simulink model "LQR_ACC_Current"  (R2024a)
settings: Solver=FixedStepAuto  StartTime=0  StopTime=1000  FixedStep=0.05  RelTol=1e-3
undefined symbols (not defined in the file or in its folder): acc_max, acc_min, Defined, driver_set_speed, Ego, jerk_lim, K_derr, K_vh, Lane, matlabshared, preview_time_AEB, preview_time_set_spd, rel_vel_thresh, rho, simStepSize, User
libraries: roadrunnerscenario x4, dsa_UDP_Blockset x2, drivingscenarioandsensors x1, autolibshared x1
settings Model: PacingRate=10  Creator=darkh  LastModifiedBy=darkh
settings DataIOCC: ReturnWorkspaceOutputsName=sltest_internal_rrSimulationOutputVariable
settings DebuggingCC: AlgebraicLoopMsg=none
settings RTWCC: GPUComputeCapability=3.5
settings ConfigComp: CovSaveName=sltest_covdata  CovMetricSettings=dcmwe  CovEnableCumulative=off  CovSaveSingleToWorkspaceVar=on  CovSaveOutputData=off

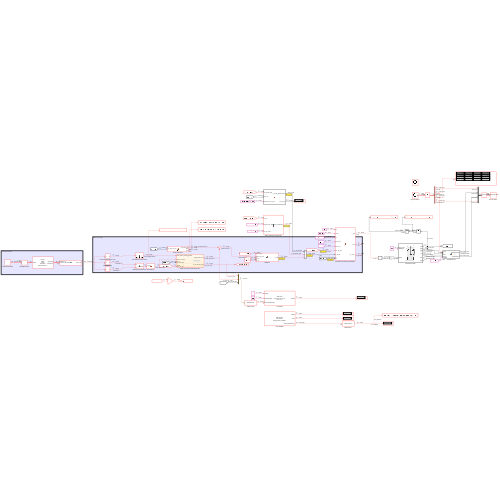
[thumbnail: Simulink's stored preview of the top-level diagram]
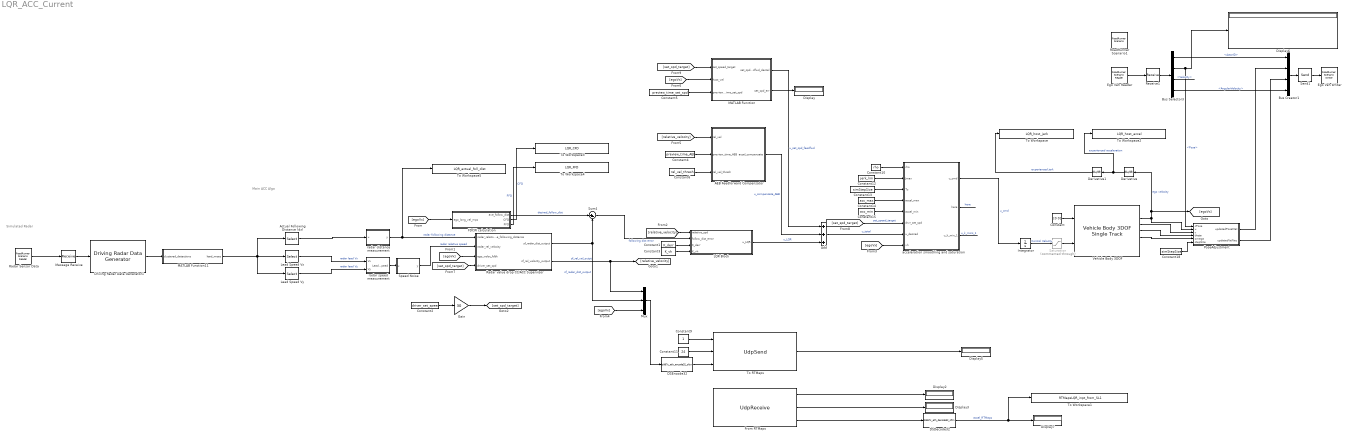
== system LQR_ACC_Current ==
  note: Simulated Radar
  note: Main ACC Algo
  AEB Feedforward Compensator : MATLAB Function  TreatAsAtomicUnit=on
  Actual Following Distance (dx) : Selector  InputPortWidth=6  IndexOptions=Index vector (dialog)  Indices=[1]  OutputSizes=1
  Add : Sum  Inputs=+++
  Bus Creator1 : BusCreator  Inputs=4  OutDataTypeStr=Bus: BusActorRuntime  NonVirtualBus=on
      settings: InheritFromInputs=off
  Bus Selector3 : BusSelector  OutputSignals=ActorID,Pose,Velocity,AngularVelocity
  Constant : Constant  Value=[0 0]
  Constant1 : Constant  Value=K_derr  SampleTime=simStepSize
  Constant10 : Constant  Value=rho
  Constant11 : Constant  Value=24
  Constant12 : Constant  Value=jerk_lim
  Constant13 : Constant  Value=simStepSize
  Constant14 : Constant  Value=acc_max
  Constant15 : Constant  Value=acc_min
  Constant18 : Constant  Value=simStepSize
  Constant2 : Constant  Value=driver_set_speed  SampleTime=simStepSize
  Constant3 : Constant  Value=K_vh  SampleTime=simStepSize
  Constant4 : Constant  Value=preview_time_AEB
  Constant5 : Constant  Value=preview_time_set_spd
  Constant6 : Constant  Value=rel_vel_thresh
  Constant9 : Constant
  "DSDecode32 " : S-Function  FunctionName=ds867c_eth_decode32_sfcn  Parameters=byteordering,offset,auto_offset,datatype,one_datatype,sampletime  SFunctionDeploymentMode=off  EnableBusSupport=off  mask(DSDecode32){byteordering=big endian (Motorola), offset=[0], auto_offset=on, datatype=[9], one_datatype=off, sampletime=-1}
      mask prompts: byteordering "Byte ordering:"; offset "Offset (bytes):"; auto_offset "Auto offset"; one_datatype "One datatype only"
      mask help:
      | Converts a 32bit WORD input data stream into the specified datatypes on the output port.
      |
      | Datatype Codes:
      | BOOLEAN:  1   //   INT8      :  2    //   UINT8    :  3
      | INT16       :  4   //   UINT16 :  5    //   INT32     :  6
      | UINT32    :  7   //   FLOAT   :  8    //   DOUBLE:  9
      mask Help:
      | The 'DSDecode32' block allows to decode an UInt32 vector containing encoded elements of various data types to an output vector of double values. It is intended to use this block in conjunction with the 'DS4504_ETH_Receive' block which delivers this format as data output. Data received from the Ethernet via the 'DS4504_ETH_Receive' block is performed in Intel byte order ('Little Endian').
      | 
      | <br>
      | <br>
      | 
      | <h2>Parameters</h2>
      | <br>
      | <br>
      | 
      | <b>Byte ordering (only relevant for offline simulation)</b>
      | <br>
      | <blockquote>
      | The byte order of the input vector has to be specified. In case of running a real-time application the appropriate byte order (Motorola for DS1005 and Intel for DS1006) is selected automatically. Therefore the byte order setting has no influence on the online simulation.
      | </blockquote>
      | <br>
      | 
      | <b>Offset (bytes)</b>
      | <br>
      | <blockquote>
      | This is for defining a vector of offsets which specifies the position of each element within the input vector. The offsets must be entered as an array (e.g. [1 10 . 50 54] ) using the same order as for the corresponding data type vector (see (4)). This option is useful if you have gaps between adjacent elements.
      | </blockquote>
      | <br>
      | 
      | <b>Auto offset</b>
      | <br>
      | <blockquote>
      | When activating this checkbox parameter, the edit field 'Offset' is disabled and the byte offsets in the input vector are calculated automatically concerning the specified data types (no gaps presupposed). Any previous setting in the offset vector would be ignored.
      | </blockquote>
      | <br>
      | 
      | <b>Datatype</b>
      | <br>
      | <blockquote>
      | This is for defining a vector of data types which specifies the type for each element in the input vector. Supported data types are Boolean, Int8, UInt8, Int16, UInt16, Int32, UInt32, Float and Double, which are determined by using the corresponding data type codes shown in the following table:
      | <br>
      | <br>
      | <table BORDER=1 ALIGN="center">
      | <TR>
      | <TH WIDTH=20%>Data type</TH>
      | <TH WIDTH=20%>Data type code</TH>
      | <TH WIDTH=20%>Length in bytes</TH>
      | </TR>
      | <TR><TD>Boolean</TD><TD ALIGN="center">1</TD><TD ALIGN="center">1</TD></TR>
      | <TR><TD>Int8</TD><TD ALIGN="center">2</TD><TD ALIGN="center">1</TD></TR>
      | <TR><TD>Uint8</TD><TD ALIGN="center">3</TD><TD ALIGN="center">1</TD></TR>
      | <TR><TD>Int16</TD><TD ALIGN="center">4</TD><TD ALIGN="center">2</TD></TR>
      | <TR><TD>Uint16</TD><TD ALIGN="center">5</TD><TD ALIGN="center">2</TD></TR>
      | <TR><TD>Int32</TD><TD ALIGN="center">6</TD><TD ALIGN="center">4</TD></TR>
      | <TR><TD>Uint32</TD><TD ALIGN="center">7</TD><TD ALIGN="center">4</TD></TR>
      | <TR><TD>Float</TD><TD ALIGN="center">8</TD><TD ALIGN="center">4</TD></TR>
      | <TR><TD>Double</TD><TD ALIGN="center">9</TD><TD ALIGN="center">8</TD></TR>
      | </TABLE>
      | </blockquote>
      | <br>
      | 
      | <b>One datatype only</b>
      | <br>
      | <blockquote>
      | This option is useful if all elements of the input vector have the same data type. If the checkbox is activated the first element of the data type vector specifies the data type to be used. In this case it is naturally sufficient to enter only one number which applies for the complete input vector.
      | </blockquote>
      | <br>
      | 
      | <b>Sample time</b>
      | <br>
      | <blockquote>
      | The desired sample time for this block has to be entered here. Alternatively it can be  inherited from the Simulink model by using '-1'.
      | </blockquote>
      | <br>
      mask TypeOptions byteordering: big endian (Motorola) | little endian (Intel)
      mask Display: text(0.5,0.5,'DSDecode32','HorizontalAlignment','center')
  DSEncode32 : S-Function  FunctionName=ds867c_eth_encode32_sfcn  Parameters=byteordering,offset,auto_offset,datatype,one_datatype,sampletime  SFunctionDeploymentMode=off  EnableBusSupport=off  mask(DSEncode32){byteordering=big endian (Motorola), offset=[ 0 ], auto_offset=on, datatype=[9,9,9], one_datatype=off, sampletime=-1}
      mask prompts: byteordering "Byte ordering:"; offset "Offset (bytes):"; auto_offset "Auto offset"; one_datatype "One datatype only"
      mask help:
      | Converts an input signal consisting of datatypes into a 32Bit WORD data stream on the output port.
      |
      | Datatype Codes:
      | BOOLEAN:  1   //   INT8      :  2    //   UINT8    :  3
      | INT16       :  4   //   UINT16 :  5    //   INT32     :  6
      | UINT32    :  7   //   FLOAT   :  8    //   DOUBLE:  9
      mask Help:
      | The 'DSEncode32' block is responsible for converting the input vector consisting of double values to different data types (multi-byte numbers) and merging them into a data stream composed of an array of UInt32 variables. It is intended to use this block in conjunction with the 'DS4504_ETH_Send' block which delivers the data in Intel byte order to the network.
      | 
      | <br>
      | <br>
      | 
      | <h2>Parameters</h2>
      | <br>
      | <br>
      | 
      | <b>Byte ordering (only relevant for offline simulation)</b>
      | <br>
      | <blockquote>
      | It lets the user choose the byte order (Motorola or Intel) of the output vector. The way multibyte numbers (e.g. Float = 4 bytes or Int16 = 2 bytes) are stored in memory depends on the used computing system. There are two possible formats which are called "Little Endian" and "Big Endian". "Little Endian" means that the low-order byte of the number is stored at the lowest and the high-order byte at the highest memory address. "Big Endian" means the opposite.
      | This option is only relevant for offline (Simulink) simulation. In case of running a real-time application the appropriate byte order (Motorola for DS1005 and Intel for DS1006) is selected automatically. Therefore the byte order setting has no influence on the online simulation.
      | </blockquote>
      | <br>
      | 
      | <b>Offset (bytes)</b>
      | <br>
      | <blockquote>
      | This is for defining a vector of offsets which specifies the position of each input element within the output byte vector. The offsets must be entered as an array (e.g. [1 10 . 50 54] ) using the same order as for the corresponding data type vector (see (4)). This option is useful if you want to have gaps between adjacent elements (e.g. in order to avoid access to even bytes).
      | <br>
      | <br>
      | <i>Important Note:</i>
      | <br>
      | By means of the offset vector the specified data values can be located flexibly within the UInt32 word stream, presupposed that the data values do not overlap. Otherwise data loss occurs.
      | </blockquote>
      | <br>
      | 
      | <b>Auto offset</b>
      | <br>
      | <blockquote>
      | When activating this checkbox parameter, the edit field 'Offset' is disabled and the required byte offsets for the input data types will be calculated automatically without gaps (for tight packing). This option is always useful if there is no need for special offsets (no gaps between two adjacent elements). Any previous setting in the offset vector would be ignored.
      | </blockquote>
      | <br>
      | 
      | <b>Datatype</b>
      | <br>
      | <blockquote>
      | This is for defining a vector of data types which specifies the type for each input element in the output byte vector. Supported data types are Boolean, Int8, UInt8, Int16, UInt16, Int32, UInt32, Float and Double, which are determined by using the corresponding data type codes shown in the following table:
      | <br>
      | <br>
      | <table BORDER=1 ALIGN="center">
      | <TR>
      | <TH WIDTH=20%>Data type</TH>
      | <TH WIDTH=20%>Data type code</TH>
      | <TH WIDTH=20%>Length in bytes</TH>
      | </TR>
      | <TR><TD>Boolean</TD><TD ALIGN="center">1</TD><TD ALIGN="center">1</TD></TR>
      | <TR><TD>Int8</TD><TD ALIGN="center">2</TD><TD ALIGN="center">1</TD></TR>
      | <TR><TD>Uint8</TD><TD ALIGN="center">3</TD><TD ALIGN="center">1</TD></TR>
      | <TR><TD>Int16</TD><TD ALIGN="center">4</TD><TD ALIGN="center">2</TD></TR>
      | <TR><TD>Uint16</TD><TD ALIGN="center">5</TD><TD ALIGN="center">2</TD></TR>
      | <TR><TD>Int32</TD><TD ALIGN="center">6</TD><TD ALIGN="center">4</TD></TR>
      | <TR><TD>Uint32</TD><TD ALIGN="center">7</TD><TD ALIGN="center">4</TD></TR>
      | <TR><TD>Float</TD><TD ALIGN="center">8</TD><TD ALIGN="center">4</TD></TR>
      | <TR><TD>Double</TD><TD ALIGN="center">9</TD><TD ALIGN="center">8</TD></TR>
      | </TABLE>
      | </blockquote>
      | <br>
      | 
      | <b>One datatype only</b>
      | <br>
      | <blockquote>
      | This option is useful if all elements of the data input vector shall be converted to the same data type in the output vector. If the checkbox is activated the first element of the data type vector specifies the data type to be used. In this case it is naturally sufficient to enter only one number which applies for the complete input vector.
      | </blockquote>
      | <br>
      | 
      | <b>Sample time</b>
      | <br>
      | <blockquote>
      | The desired sample time for this block has to be entered here. Alternatively it can be  inherited from the Simulink model by using '-1'.
      | </blockquote>
      | <br>
      mask TypeOptions byteordering: big endian (Motorola) | little endian (Intel)
      mask Display: text(0.5,0.5,'DSEncode32','HorizontalAlignment','center')
  Derivative : Derivative
  Derivative1 : Derivative
  Display{,2..3,5..7} (6 alike) : Display
  Driving Radar Data Generator1 : drivingscenarioandsensors/Driving Radar Data Generator  SensorIndex=1  UpdateRate=20  MountingLocation=[ 3.4, 0, 0.2 ]  MountingAngles=[0 0 0]  HasElevation=off  HasRangeRate=on  HasNoise=off  HasFalseAlarms=off  HasOcclusion=off  MaxNumReportsSource=Property  MaxNumReports=50  TargetReportFormat=Clustered detections  DetectionCoordinates=Body  TrackCoordinates=Body  BusNameSource=Auto  BusName=BusDrivingRadarDataGenerator  AzimuthResolution=4  ElevationResolution=5  RangeResolution=2.5  RangeRateResolution=0.05  AzimuthBiasFraction=0.1  ElevationBiasFraction=0.1  RangeBiasFraction=0.01  RangeRateBiasFraction=0.01  FieldOfView=[ 20, 5 ]  RangeLimits=[ 0, 150 ]  RangeRateLimits=[ -100, 100 ]  DetectionProbability=1  FalseAlarmRate=1e-06  ReferenceRange=100  ReferenceRCS=0  CenterFrequency=77e9  FilterInitializationFcn=initcvekf  ConfirmationThreshold=[2 3]  DeletionThreshold=[5 5]  InitialSeedSource=Repeatable  InitialSeed=0  UsedSeed=matlabshared.tracking.internal.SimulinkUtilities.seedManager(gcb)  ProfilesSource=From Scenario Reader block  ProfilesParameters=driving.internal.ActorProfilesRadarParameters  ProfilesExpression=struct('ClassID',0,'Length',4.7,'Width',1.8,'Height',1.4,'OriginOffset',[-1.35 0 0],'RCSPattern',[10 10;10 10],'RCSAzimuthAngles',[-180 180],'RCSElevationAngles',[-90 90])
  Ego Veh Reader : roadrunnerscenario/RoadRunner Scenario Reader  TopicCategory=Actor  ActorCategory=All Types  ActionType=Path Following  EventType=User-Defined  TopicType=Actor Pose  VehicleType=Vehicle Specifications  UserDefinedAction=Action1  UserDefinedEvent=Event1  Filter=Self  SensorTopic=Target Poses  LaneBoundaryOutputTopic=Ego-Lane  SensorID=1  SampleTime=simStepSize
  Ego Veh Writer : roadrunnerscenario/RoadRunner Scenario Writer  TopicCategory=Actor  ActorCategory=All Types  EventType=Action Complete  UserDefinedEvent=Event1  VehicleType=Vehicle Pose  TopicType=Actor Pose
  FDCW calculation : MATLAB Function  TreatAsAtomicUnit=on
  From RTMaps : dsa_UDP_Blockset/UdpReceive  portNumber=25000  sampleTime=simStepSize  outputWidth=1472  rxTimeout=1  rxBufferSize=73600
  Gain : Gain  Gain=30
  Integrator : Integrator
  LQR Block : MATLAB Function  TreatAsAtomicUnit=on  SystemSampleTime=simStepSize
  Lead Speed Vx : Selector  InputPortWidth=6  IndexOptions=Index vector (dialog)  Indices=4  OutputSizes=1
  Lead Speed Vy : Selector  InputPortWidth=6  IndexOptions=Index vector (dialog)  Indices=5  OutputSizes=1
  MATLAB Function : MATLAB Function  TreatAsAtomicUnit=on
  MATLAB Function11 : MATLAB Function  TreatAsAtomicUnit=on
  Message Receive : Receive  InputPortMessageModes=m  UseInternalQueue=off
  Mux : Mux  Inputs=3
  PoseAdjustment : MATLAB Function  TreatAsAtomicUnit=on
  Radar Sensor Data : roadrunnerscenario/RoadRunner Scenario Reader  TopicCategory=Sensor  ActorCategory=All Types  ActionType=Path Following  EventType=User-Defined  TopicType=Actor Specifications  VehicleType=Vehicle Specifications  UserDefinedAction=Action1  UserDefinedEvent=Event1  Filter=Self  SensorTopic=Target Poses  LaneBoundaryOutputTopic=Ego-Lane  SensorID=1  SampleTime=simStepSize
  Radar value drop CC/ACC Supervisor : Stateflow chart  TreatAsAtomicUnit=on
  Receive1 : Receive  InputPortMessageModes=m  UseInternalQueue=off  QueueOverwriting=on  QueueLength=1  QueueType=LIFO
  RoadRunner Scenario1 : roadrunnerscenario/RoadRunner Scenario  UserDefinedActions={}  UserDefinedEvents={}
  Saturation : Saturate  Commented=through  UpperLimit=driver_set_speed  LowerLimit=0
  Send1 : Send  OutputPortMessageModes=m
  Speed Noise : MATLAB Function  TreatAsAtomicUnit=on
  Sum4 : Sum  Inputs=|+-
  To RTMaps : dsa_UDP_Blockset/UdpSend  hostName=192.168.140.10  portNumber=11111
  To Workspace : ToWorkspace  VariableName=LQR_host_jerk  SampleTime=-1
  To Workspace1 : ToWorkspace  VariableName=RTMapsLQR_inpt_from_SL1  SaveFormat=Timeseries  SampleTime=-1
  To Workspace2 : ToWorkspace  VariableName=LQR_host_accel  SampleTime=-1
  To Workspace3 : ToWorkspace  VariableName=LQR_CFD  SampleTime=-1
  To Workspace4 : ToWorkspace  VariableName=LQR_FFD  SampleTime=-1
  To Workspace5 : ToWorkspace  VariableName=LQR_actual_foll_dist  SampleTime=-1
  "Vehicle Body 3DOF " : autolibshared/Vehicle Body 3DOF Single Track  trackMode=Dual  inputMode=External longitudinal velocity  frontSteerMode=on  rearSteerMode=off  windMode=off  muMode=off  extFMode=off  extMMode=off  htchFMode=off  htchMMode=off  extXo=off  extpsio=off  extxdoto=off  extro=off  extYo=off  extTamb=off  extydoto=off  aMode=2  NF=2  NR=2  m=2630.84  a=1.5569  b=1.5371  h=0.18903  dh=1  hh=0.2  X_o=0  xdot_o=0  CalphaMode=off  sigmaMode=on  d=0  hl=0  w=[1.4,1.4]  Cy_f=40000  Cy_r=40000  sigma_f=.1  sigma_r=.1  alpha_f_brk=[-.1 .1]  Cy_f_data=[-9e3 9e3]  alpha_r_brk=[-.1 .1]  Cy_r_data=[-9e3 9e3]  Y_o=0  ydot_o=0  Izz=2066  psi_o=0  r_o=0  Af=2.73  Cd=.30356  Cl=.1  Cpm=.1  beta_w=[0 0.01:0.01:0.3]  Cs=[0 0.01:0.01:0.3]  Cym=[0 1e-6:0.01:0.3]  Pabs=101325  Tair=273  g=9.81  mu=1  xdot_tol=.01  Fznom=5000  Fxtire_sat=7e4  Fytire_sat=7e4  longOff=0  latOff=0  vertOff=0  wrapAng=off
  acceleration smoothing and saturation : MATLAB Function  TreatAsAtomicUnit=on  SystemSampleTime=simStepSize
  radar distance measurement : MATLAB Function  TreatAsAtomicUnit=on
  radar speed measurement : MATLAB Function  TreatAsAtomicUnit=on
  wires:
  Bus Selector3/4 -> Bus Creator1/4  "<AngularVelocity>"
  Bus Creator1/1 -> Send1/1
  Bus Selector3/1 -> Bus Creator1/1  "<ActorID>"
  Receive1/1 -> Bus Selector3/1
  Send1/1 -> Ego Veh Writer/1
  Ego Veh Reader/1 -> Receive1/1
  "Vehicle Body 3DOF "/3 -> PoseAdjustment/3(v)
  "Vehicle Body 3DOF "/4 -> PoseAdjustment/4(theta)
  "Vehicle Body 3DOF "/5 -> PoseAdjustment/5(omega)
  Bus Selector3/2 -> Display6/1, PoseAdjustment/1(cPose)  "<Pose>"
  PoseAdjustment/1(updatedPoseMat) -> Bus Creator1/2
  "Vehicle Body 3DOF "/2 -> PoseAdjustment/2(u), Derivative/1, [egoVx]  "ego velocity"
  Radar Sensor Data/1 -> Message Receive/1
  Message Receive/1 -> Driving Radar Data Generator1/1
  Driving Radar Data Generator1/1 -> MATLAB Function11/1(clustered_detections)
  PoseAdjustment/2(updatedVelVec) -> Bus Creator1/3
  Integrator/1 -> Saturation/1  "Control Velocity"
  Constant/1 -> "Vehicle Body 3DOF "/1
  Sum4/1 -> LQR Block/2(follow_dist_error)  "following dist error"
  Constant1/1 -> LQR Block/3(K_derr)
  Lead Speed Vx/1 -> radar speed measurement/1(Vx)  "radar lead Vx"
  [egoVx] -> FDCW calculation/1(ego_long_vel_mps)
  FDCW calculation/1(ave_follow_dist) -> Sum4/1  "desired_follow_dist"
  MATLAB Function11/1(lead_meas) -> Actual Following Distance (dx)/1, Lead Speed Vy/1, Lead Speed Vx/1
  Lead Speed Vy/1 -> radar speed measurement/2(Vy)  "radar lead Vy"
  radar speed measurement/1(LeadSpeed) -> Speed Noise/1(u)
  FDCW calculation/2(CFD) -> To Workspace3/1  "CFD"
  Actual Following Distance (dx)/1 -> radar distance measurement/1(u)
  Derivative/1 -> To Workspace2/1, Derivative1/1  "experienced acceleration"
  Derivative1/1 -> To Workspace/1  "experienced jerk"
  [egoVx] -> Radar value drop CC/ACC Supervisor/3(ego_veloc_fdbk)
  Constant2/1 -> Gain/1
  Speed Noise/1(y) -> Radar value drop CC/ACC Supervisor/2(radar_rel_velocity)  "radar relative speed"
  radar distance measurement/1(y) -> To Workspace5/1, Radar value drop CC/ACC Supervisor/1(radar_relative_following_distance)  "radar following distance"
  Radar value drop CC/ACC Supervisor/1(sf_radar_dist_output) -> Mux/2, Sum4/2  "sf_radar_dist_output"
  Radar value drop CC/ACC Supervisor/2(sf_rel_velocity_output) -> Mux/1, [relative_velocity]  "sf_rel_vel_outpt"
  Constant3/1 -> LQR Block/4(K_vh)
  Mux/1 -> DSEncode32/1
  Constant9/1 -> To RTMaps/1
  Constant11/1 -> To RTMaps/2
  To RTMaps/1 -> Display5/1
  From RTMaps/1 -> Display2/1
  From RTMaps/2 -> Display3/1
  From RTMaps/3 -> "DSDecode32 "/1
  DSEncode32/1 -> To RTMaps/3
  "DSDecode32 "/1 -> Display7/1, To Workspace1/1  "accel_RTMaps"
  LQR Block/1(u_LQR) -> Add/3  "u_LQR"
  Constant12/1 -> acceleration smoothing and saturation/2(Jmax)
  Constant13/1 -> acceleration smoothing and saturation/3(Ts)
  Constant14/1 -> acceleration smoothing and saturation/4(accel_max)
  Constant15/1 -> acceleration smoothing and saturation/5(accel_min)
  Constant10/1 -> acceleration smoothing and saturation/1(rho)
  [egoVx] -> acceleration smoothing and saturation/8(vh)
  [set_spd_target] -> acceleration smoothing and saturation/6(drvr_set_spd)  "set_speed_target"
  Bus Selector3/3 -> ?  "<Velocity>"
  Saturation/1 -> "Vehicle Body 3DOF "/2
  [egoVx] -> Mux/3
  FDCW calculation/3(FFD) -> To Workspace4/1  "FFD"
  acceleration smoothing and saturation/1(u_cmd) -> Integrator/1  "u_cmd"
  Constant18/1 -> PoseAdjustment/6(stepSize)
  [relative_velocity] -> LQR Block/1(relative_spd)
  [relative_velocity] -> AEB Feedforward Compensator/1(rel_vel)
  Constant4/1 -> AEB Feedforward Compensator/2(preview_time_AEB)
  Constant6/1 -> AEB Feedforward Compensator/3(rel_vel_thresh)
  AEB Feedforward Compensator/1(accel_compensate) -> Add/2  "u_compensate_AEB"
  Add/1 -> acceleration smoothing and saturation/7(u_desired)  "u_total"
  MATLAB Function/2(set_spd_err) -> Display/1
  [egoVx] -> MATLAB Function/2(host_vel)
  Constant5/1 -> MATLAB Function/3(preview_time_set_spd)
  MATLAB Function/1(set_spd_feedfwd_deccel) -> Add/1  "u_set_spd_feedfwd"
  [set_spd_target] -> Radar value drop CC/ACC Supervisor/4(driver_set_spd)
  [set_spd_target] -> MATLAB Function/1(set_speed_target)
  Gain/1 -> [set_spd_target]
  acceleration smoothing and saturation/2(here) -> ?  "here"
  acceleration smoothing and saturation/3(u_k_min_1) -> ?  "u_k_mins_1"

== matlab function LQR_ACC_Current/radar distance measurement ==
  data: u input; y output
function y = removeSpikes(u)

    persistent buffer;
    persistent bufferIndex;
    threshold = 2;
    windowSize = 15;
    % windowSize = 4;
    
    if isempty(buffer)
        buffer = zeros(1, windowSize);
        bufferIndex = 1;
    end
    
    % Update buffer with new value
    buffer(bufferIndex) = u;
    bufferIndex = mod(bufferIndex, windowSize) + 1;
    
    % Calculate the median of the buffer
    medVal = median(buffer);
    
    % Detect and remove spikes
    if abs(u - medVal) > threshold
        y = medVal; % Replace spike with the median value
    else
        y = u; % Keep the original value if it's not a spike
    end
end

== matlab function LQR_ACC_Current/radar speed measurement ==
  data: Vx input; LeadSpeed output; Vy input
function LeadSpeed = fcn(Vx, Vy)

if Vx == 0 && Vy == 0 
    Vx = 0.01;
    Vy = 0.01;
elseif Vy == 0
    Vy = 0.01;
elseif Vx == 0
    Vx = 0.01;
end

if Vx <= 0
    LeadSpeed = -sqrt(Vx^2 + Vy^2);
else
    LeadSpeed = sqrt(Vx^2 + Vy^2);
end

== matlab function LQR_ACC_Current/Speed Noise ==
  settings: updateMethod=DISCRETE
  data: u input; y output
function y = removeSpikes(u)
    % removeSpikes - Removes spikes from a scalar signal based on a threshold
    %
    % Inputs:
    %    u - The input signal (scalar)
    %    threshold - The threshold value to detect spikes
    %    windowSize - The size of the window for calculating the median
    %
    % Outputs:
    %    y - The filtered signal with spikes removed

    % Declare persistent variables to store past values
    persistent buffer;
    persistent bufferIndex;
    threshold = 2;
    windowSize = 15;
    % windowSize = 5;

    
    if isempty(buffer)
        buffer = zeros(1, windowSize);
        bufferIndex = 1;
    end
    
    % Update buffer with new value
    buffer(bufferIndex) = u;
    bufferIndex = mod(bufferIndex, windowSize) + 1;
    
    % Calculate the median of the buffer
    medVal = median(buffer);
    
    % Detect and remove spikes
    if abs(u - medVal) > threshold
        y = medVal; % Replace spike with the median value
    else
        y = u; % Keep the original value if it's not a spike
    end
end

== matlab function LQR_ACC_Current/MATLAB Function11 ==
  data: clustered_detections input Bus: BusRadar; lead_meas output double
function lead_meas = fcn(clustered_detections)

lead_det = clustered_detections.Detections(1);
lead_meas = lead_det.Measurement;

% relative_dist = sqrt(lead_det.Measurement(1)^2 + lead_det.Measurement(2)^2); % rel_dist = sqrt(x^2+y^2)
% relative_speed = sqrt(lead_det.Measurement(4)^2 + lead_det.Measurement(5)^2);
end

== matlab function LQR_ACC_Current/FDCW calculation ==
  settings: updateMethod=DISCRETE
  data: ego_long_vel_mps input; ave_follow_dist output; CFD output; FFD output
% Function to determine the closest (CFD) and furthest follow distance (FFD) for the
% ego vehicle relative to the lead vehicle given the ego vehicle's current
% velocity

% This function outputs the middle distance value between the CFD and FFD
% and those values respectively as well

function [ave_follow_dist, CFD, FFD] = fcn(ego_long_vel_mps)
    persistent dist_history window_size smoothing_weights
    
    % Initialize (first call only)
    if isempty(dist_history)
        window_size = 5;  % Number of past samples
        dist_history = zeros(1, window_size);
        
        % Define and normalize weights (e.g., linear decay)
        smoothing_weights = linspace(1, 0.5, window_size);  % Weights from 1.0 to 0.5
        smoothing_weights = smoothing_weights / sum(smoothing_weights);  % Normalize
    end
    
    ego_long_vel_mph = ego_long_vel_mps*2.23694; % from metres per secs to miles per hour

    if ego_long_vel_mph > 0 && ego_long_vel_mph < 20
        CFD = 2.8*ego_long_vel_mph^0.45+8;
        FFD = 100-0.2*(20-ego_long_vel_mph)^2;
    elseif ego_long_vel_mph <= 0
        CFD = 8;
        FFD = 100-0.2*(20)^2;
    else
        CFD = 2.8*ego_long_vel_mph^0.45+8;
        FFD = 100;
    end
    AveFollowDist_Gain = 2;


    % --- Update history buffer ---
    dist_history = [ ((AveFollowDist_Gain-1)*CFD + FFD)/AveFollowDist_Gain , dist_history(1:end-1)];  % FIFO

    % --- Smoothed average (weighted, normalized) ---
    smoothed_ave_dist = sum(dist_history .* smoothing_weights);
    
    % --- Clamp to CFD/FFD bounds ---
    ave_follow_dist = min(max(smoothed_ave_dist, CFD), FFD);
end

== matlab function LQR_ACC_Current/LQR Block ==
  data: relative_spd input; u_LQR output; follow_dist_error input; K_derr input; K_vh input
function u_LQR = fcn(relative_spd, follow_dist_error, K_derr, K_vh)
u_LQR = -K_derr*follow_dist_error-K_vh*relative_spd;

== matlab function LQR_ACC_Current/AEB Feedforward Compensator ==
  data: rel_vel input; accel_compensate output; preview_time_AEB input; rel_vel_thresh input
function accel_compensate = fcn(rel_vel, preview_time_AEB, rel_vel_thresh)
% This function determines a feedforward decceleration to apply to vehicle
% in the event that the vehicle approaches a stopped car at high speed,
% i.e. Automatic Emergency Braking (AEB) event
% rel_vel is the relative velocity compared to lead vehicle [m/s]; 
% preview_time is the time in [secs] over which the car should slow down based on the relative velocity; 
% rel_vel_thresh is the relative velocity threshold, smaller relative velocity differences than this value will be ignored [m/s]

if rel_vel > -rel_vel_thresh
    accel_compensate = 0.0;
    return;
end

accel_compensate = rel_vel/preview_time_AEB;

== stateflow chart LQR_ACC_Current/Radar value drop CC//ACC Supervisor ==
  state Radar_State_Lead_Veh_Present_and_Detected
    sf_radar_dist_output = radar_relative_following_distance;
    sf_rel_velocity_output = radar_rel_velocity;
    counter = counter + 1; % updates by 1 every time step; to wait to give the radar time to initialize in simulation
  state Output_Spoof_To_Keep_Moving
    %sf_radar_dist_output = 150;
    sf_radar_dist_output = smooth_switch(sf_radar_dist_output, 70, 0.05, 2);
    set_spd_err = driver_set_spd - ego_veloc_fdbk;
    sf_rel_velocity_output = set_spd_err;
    % sf_rel_velocity_output = smooth_switch(sf_rel_velocity_output, set_spd_err, 0.05, 5);
  (default) -> Radar_State_Lead_Veh_Present_and_Detected : {sf_radar_dist_output = radar_relative_following_distance;
      | sf_rel_velocity_output = radar_rel_velocity;
      | counter = 0;}
  Radar_State_Lead_Veh_Present_and_Detected -> Output_Spoof_To_Keep_Moving : [radar_relative_following_distance == 0 && radar_rel_velocity < 0.9 && counter > 3]
  Output_Spoof_To_Keep_Moving -> Radar_State_Lead_Veh_Present_and_Detected : [radar_relative_following_distance > 0]
  data: prev_val function_input; curr_val function_input; dt function_input; tau function_input; filtered_val function_output; radar_relative_following_distance input; sf_radar_dist_output output; radar_rel_velocity input; ego_veloc_fdbk input; sf_rel_velocity_output output; driver_set_spd input; set_spd_err local; counter local
  function filtered_val = smooth_switch(prev_val, curr_val, dt, tau):
    | function filtered_val = smooth_switch(prev_val, curr_val, dt, tau)
    | % Smooth transition from prev_val toward curr_val
    | % dt  = sample time [s]; equal to system sample time of 0.05s currently
    | % tau = time constant [s] (0.3–1.0 typical)
    | 
    | if isempty(prev_val)
    |     prev_val = 0;
    | end
    | 
    | alpha = exp(-dt/tau);
    | filtered_val = alpha*prev_val + (1-alpha)*curr_val;
    | end

== matlab function LQR_ACC_Current/acceleration smoothing and saturation ==
  data: rho input; Jmax input; Ts input; accel_max input; accel_min input; drvr_set_spd input; u_cmd output; u_desired input; vh input; here output; u_k_min_1 output
function [u_cmd, here, u_k_min_1] = fcn(rho, Jmax, Ts, accel_max, accel_min, drvr_set_spd, u_desired, vh)
% function u_cmd = fcn(rho, Jmax, Ts, accel_max, accel_min, drvr_set_spd, u_desired, vh)
% This function is the smoothing step that determines a commanded control
% signal based on minimizing the following QP : J(u) = (u-u_lqr)^2 + rho*(u - uk_minus_1)^2
% This block also limits the acceleration output if the vehicle is at or past the driver set speed value OR if telling car to go backwards

persistent u_k_minus_1
if isempty(u_k_minus_1)
    u_k_minus_1 = 0.0;
end

u_k_min_1 = u_k_minus_1; % for debugginggggggg

u_tilde = (u_desired + rho*u_k_minus_1)/(1 + rho); % jerk and control deviation cost minimizing control signal

u_cmd = min(max(u_tilde, u_k_minus_1 - Jmax*Ts), u_k_minus_1 + Jmax*Ts); % rate-limiting the control signal (jerk limits)
u_cmd = min(max(u_cmd, accel_min), accel_max); % Applying acceleration magnitude limits to control signal

here = 0; % for debugging

if (vh <= 0.001 && u_cmd < 0.0) % If vehicle is at a full stop and controller requests a negative acceleration, set commanded accel to 0 m/s^2
    % alpha = exp(-Ts/0.5);
    % u_cmd = alpha*u_k_minus_1 + (1-alpha)*0.0;
    u_cmd = 0.0;
    u_k_minus_1 = u_cmd; % updating previous input value for use next timestep

    here  = 1;
    return;

elseif (vh >= drvr_set_spd-0.5 && u_cmd >= 0.0) % If vehicle is approaching driver set limit and controller requests positive accel, set command to 0 m/s^2
    % % filtered_val = alpha*prev_val + (1-alpha)*curr_val; Smooth transition from prev_val toward curr_val; where alpha = exp(-dt/tau)
    % % dt  = sample time [s]; equal to system sample time of 0.05s currently
    % % tau = time constant [s] (0.3–1.0 typical)
    % alpha = exp(-Ts/1.0);
    % u_cmd = alpha*u_k_minus_1 + (1-alpha)*0.0;
    % u_cmd = 0.0;
    
    u_cmd = min(max(0.0, u_k_minus_1 - Jmax*Ts), u_k_minus_1 + Jmax*Ts); % Move to 0.0 m/s^2 acceleration with maximum allowable jerk
    u_k_minus_1 = u_cmd; % updating previous input value for use next timestep
    
    here = 2;
    return;
end

u_k_minus_1 = u_cmd; % updating previous input value for use next timestep

== matlab function LQR_ACC_Current/MATLAB Function ==
  data: set_speed_target input; set_spd_feedfwd_deccel output; host_vel input; preview_time_set_spd input; set_spd_err output
function [set_spd_feedfwd_deccel, set_spd_err] = fcn(set_speed_target, host_vel, preview_time_set_spd)
% This function determines the feedforward slowing down effect for host if
% the vehicle ever exceeds the set speed maximum/driver set speed/speed target set by AIN feature
% inputs are set_speed_target [m/s] which is speed maximum value; host_vel which is host velocity feedback [m/s]; 
% preview_time [secs] is how quickly want vehicle to slow down to bring below/at set speed maximum

set_spd_err = set_speed_target - host_vel; % if over set speed limit this value will be negative
if set_spd_err < 0.0
    set_spd_feedfwd_deccel = set_spd_err/preview_time_set_spd;
    return;
end

set_spd_feedfwd_deccel = 0.0;

== matlab function LQR_ACC_Current/PoseAdjustment ==
  data: cPose input; u input; updatedPoseMat output; v input; theta input; omega input; updatedVelVec output; stepSize input
function [updatedPoseMat, updatedVelVec] = fcn(cPose, u, v, theta, omega, stepSize)
    thetad = theta + omega*stepSize;
    xd = (u*cos(theta) - v*sin(theta))*stepSize;
    yd = (u*sin(theta) + v*cos(theta))*stepSize;
    pose_mat = [cos(-thetad) -sin(-thetad) 0 (yd+cPose(1,4)); sin(-thetad) cos(-thetad) 0 (xd+cPose(2,4)); 0 0 1 0; 0 0 0 1];
    updatedPoseMat = pose_mat;
    updatedVelVec = [u*sin(theta) + v*cos(theta), u*cos(theta) - v*sin(theta), 0];
    return;
end
